simulink model "fu_simu_png_radome"  (R2020a)
settings: Solver=FixedStepAuto  StartTime=0.0  StopTime=20  FixedStep=0.001  RelTol=1e-3
values from neighbouring files (symbols this model uses):
  gamma_M_0 = deg2rad(0)    [initial.m]
  lambda_0 = deg2rad(5.7106)    [initial.m]
  lambda_r_0 = rho_0*(lambda_0-theta_M_0)    [initial.m]
  N = 4    [initial.m]
  R_0 = 10050    [initial.m]
  T_alpha = 1    [initial.m]
  tau = 0.1    [initial.m]
  V_M = 500    [initial.m]
settings Model: Creator=anwaei  LastModifiedBy=anwaei

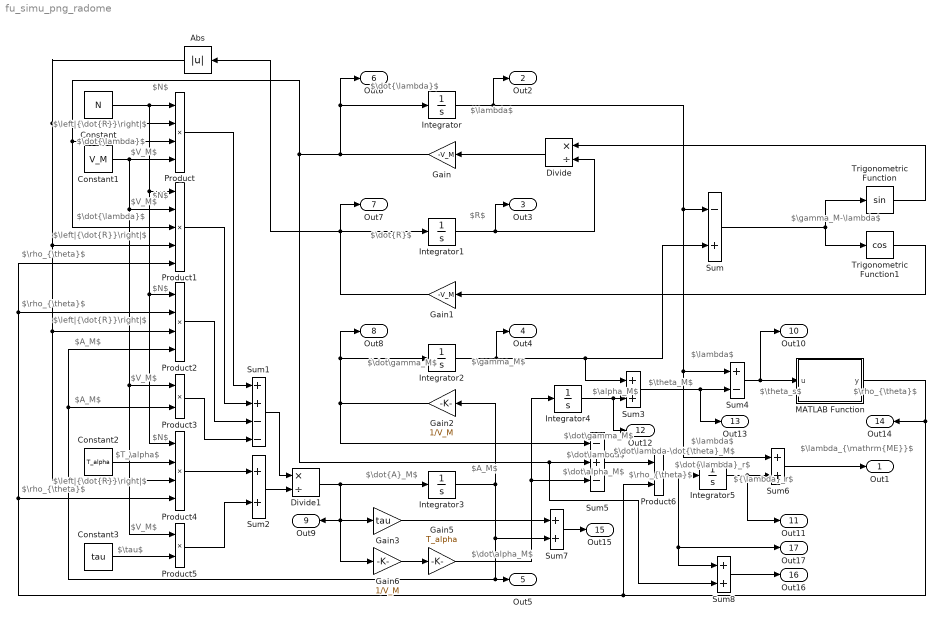
== system fu_simu_png_radome ==
  note: $\lambda$
  note: $R$
  note: $\gamma_M$
  note: $A_M$
  note: $\gamma_M-\lambda$
  note: $\dot{\lambda}$
  note: $\dot{R}$
  note: $\left|{\dot{R}}\right|$
  note: $\left|{\dot{R}}\right|$
  note: $\left|{\dot{R}}\right|$
  note: $\rho_{\theta}$
  note: $\dot{\lambda}$
  note: $\dot{\lambda}$
  note: $A_M$
  note: $A_M$
  note: $N$
  note: $N$
  note: $N$
  note: $N$
  note: $V_M$
  note: $V_M$
  note: $V_M$
  note: $V_M$
  note: $T_\alpha$
  note: $\tau$
  note: $\dot\gamma_M$
  note: $\dot{A}_M$
  note: $\alpha_M$
  note: $\theta_M$
  note: $\left|{\dot{R}}\right|$
  note: $\rho_{\theta}$
  note: $\rho_{\theta}$
  note: $\rho_{\theta}$
  note: $\theta_s$
  note: $\dot\alpha_M$
  note: $\dot\gamma_M$
  note: $\dot\lambda$
  note: $\dot\alpha_M$
  note: $\dot\lambda-\dot{\theta}_M$
  note: $\rho_{\theta}$
  note: $\dot{\lambda}_r$
  note: $\lambda$
  note: $\lambda$
  note: ${\lambda}_r$
  note: $\lambda_{\mathrm{ME}}$
  Abs : Abs
  Constant : Constant  Value=N
  Constant1 : Constant  Value=V_M
  Constant2 : Constant  Value=T_alpha
  Constant3 : Constant  Value=tau
  Divide : Product  Inputs=*/
  Divide1 : Product  Inputs=*/
  Gain : Gain  Gain=-V_M
  Gain1 : Gain  Gain=-V_M
  Gain2 : Gain  Gain=1/V_M
  Gain3 : Gain  Gain=tau
  Gain5 : Gain  Gain=T_alpha
  Gain6 : Gain  Gain=1/V_M
  Integrator : Integrator  InitialCondition=lambda_0
  Integrator1 : Integrator  InitialCondition=R_0
  Integrator2 : Integrator  InitialCondition=gamma_M_0
  Integrator3 : Integrator
  Integrator4 : Integrator
  Integrator5 : Integrator  InitialCondition=lambda_r_0
  MATLAB Function : MATLAB Function  TreatAsAtomicUnit=on
  Product : Product  Inputs=4
  Product1 : Product  Inputs=5
  Product2 : Product  Inputs=4
  Product3 : Product
  Product4 : Product  Inputs=4
  Product5 : Product
  Product6 : Product
  Sum : Sum  Inputs=-+
  Sum1 : Sum  Inputs=++--
  Sum{2..3,6..8} (5 alike) : Sum
  Sum4 : Sum  Inputs=+-
  Sum5 : Sum  Inputs=-+-
  Trigonometric Function : Trigonometry
  Trigonometric Function1 : Trigonometry  Operator=cos
  Out1 : Outport
  Out2 : Outport  Port=2
  Out3 : Outport  Port=3
  Out4 : Outport  Port=4
  Out5 : Outport  Port=5
  Out6 : Outport  Port=6
  Out7 : Outport  Port=7
  Out8 : Outport  Port=8
  Out9 : Outport  Port=9
  Out10 : Outport  Port=10
  Out11 : Outport  Port=11
  Out12 : Outport  Port=12
  Out13 : Outport  Port=13
  Out14 : Outport  Port=14
  Out15 : Outport  Port=15
  Out16 : Outport  Port=16
  Out17 : Outport  Port=17
  wires:
  Integrator/1 -> Out2/1, Sum6/1, Sum4/1, Sum/1
  Integrator1/1 -> Out3/1, Divide/2
  Integrator2/1 -> Out4/1, Sum3/1, Sum/2
  Integrator3/1 -> Gain2/1, Sum7/2, Out5/1, Product2/4, Product3/2
  Sum/1 -> Trigonometric Function/1, Trigonometric Function1/1
  Trigonometric Function/1 -> Divide/1
  Divide/1 -> Gain/1
  Gain/1 -> Sum8/2, Sum5/2, Product1/3, Product/3, Out6/1, Integrator/1
  Trigonometric Function1/1 -> Gain1/1
  Gain1/1 -> Out7/1, Abs/1, Integrator1/1
  Gain2/1 -> Sum5/1, Out8/1, Integrator2/1
  Divide1/1 -> Gain3/1, Gain6/1, Out9/1, Integrator3/1
  Sum1/1 -> Divide1/1
  Constant/1 -> Product/1, Product4/1, Product2/1, Product1/1
  Constant1/1 -> Product/4, Product1/2, Product3/1, Product5/1
  Product/1 -> Sum1/1
  Product1/1 -> Sum1/2
  Product2/1 -> Sum1/3
  Product3/1 -> Sum1/4
  Constant2/1 -> Product4/2
  Sum2/1 -> Divide1/2
  Constant3/1 -> Product5/2
  Product5/1 -> Sum2/2
  Product4/1 -> Sum2/1
  Sum3/1 -> Out13/1, Sum4/2
  Sum4/1 -> Out10/1, MATLAB Function/1(u)
  MATLAB Function/1(y) -> Out14/1, Product4/4, Product1/5, Product2/2, Product6/2
  Gain6/1 -> Gain5/1
  Gain5/1 -> Integrator4/1, Sum5/3
  Integrator4/1 -> Out12/1, Sum3/2
  Sum5/1 -> Product6/1
  Product6/1 -> Out17/1, Sum8/1, Integrator5/1
  Integrator5/1 -> Out11/1, Sum6/2
  Sum6/1 -> Out1/1
  Abs/1 -> Product4/3, Product2/3, Product1/4, Product/2
  Gain3/1 -> Sum7/1
  Sum7/1 -> Out15/1
  Sum8/1 -> Out16/1

== matlab function fu_simu_png_radome/MATLAB Function ==
  data: u input; y output
function y = fcn(u)

%%
r=-0.5;
zeta=4;
p=1;

if u<0
    a=exp(zeta*u);
    b=zeta*sin(2*pi*u/p);
    c=2*pi/p*cos(2*pi*u/p);
else
    a=exp(-zeta*u);
    b=-zeta*sin(2*pi*u/p);
    c=2*pi/p*cos(2*pi*u/p);
end

y=r*a*(b+c);
y=y/rad2deg(1);

%%
% y=0.025;
% y=0.05;
% y=-0.025;
